simulink model "full_subtractor"  (R2021a)
settings: Solver=VariableStepAuto  StartTime=0.0  StopTime=10.0  RelTol=1e-3
settings Model: Creator=kbhar  LastModifiedBy=kbhar

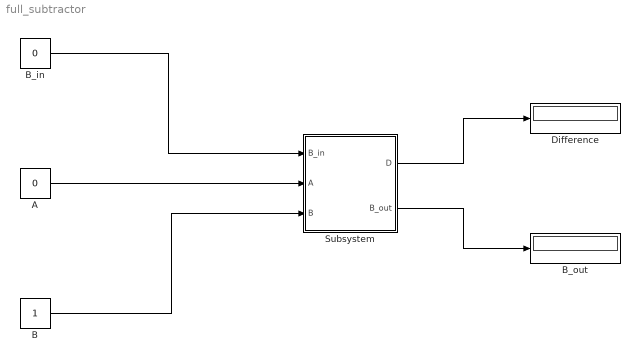
== system full_subtractor ==
  A : Constant  Value=0
  B : Constant
  B_in : Constant  Value=0
  B_out : Display
  Difference : Display
  Subsystem : Subsystem
  wires:
  B_in/1 -> Subsystem/1(B_in)
  A/1 -> Subsystem/2(A)
  B/1 -> Subsystem/3(B)
  Subsystem/1(D) -> Difference/1
  Subsystem/2(B_out) -> B_out/1

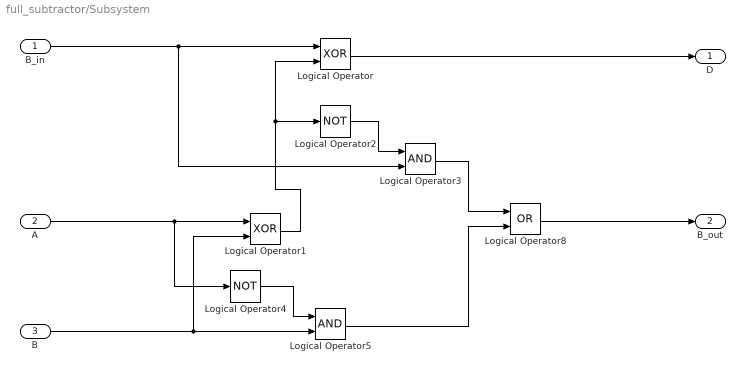
== system full_subtractor/Subsystem ==
  B_in : Inport
  A : Inport  Port=2
  B : Inport  Port=3
  Logical Operator : Logic  Operator=XOR  AllPortsSameDT=off  OutDataTypeStr=boolean
  Logical Operator1 : Logic  Operator=XOR  AllPortsSameDT=off  OutDataTypeStr=boolean
  Logical Operator2 : Logic  Operator=NOT  AllPortsSameDT=off  OutDataTypeStr=boolean
  Logical Operator3 : Logic  AllPortsSameDT=off  OutDataTypeStr=boolean
  Logical Operator4 : Logic  Operator=NOT  AllPortsSameDT=off  OutDataTypeStr=boolean
  Logical Operator5 : Logic  AllPortsSameDT=off  OutDataTypeStr=boolean
  Logical Operator8 : Logic  Operator=OR  AllPortsSameDT=off  OutDataTypeStr=boolean
  D : Outport
  B_out : Outport  Port=2
  wires:
  Logical Operator2/1 -> Logical Operator3/1
  B_in/1 -> Logical Operator/1, Logical Operator3/2
  B/1 -> Logical Operator1/2, Logical Operator5/2
  Logical Operator1/1 -> Logical Operator2/1, Logical Operator/2
  A/1 -> Logical Operator1/1, Logical Operator4/1
  Logical Operator3/1 -> Logical Operator8/1
  Logical Operator5/1 -> Logical Operator8/2
  Logical Operator4/1 -> Logical Operator5/1
  Logical Operator/1 -> D/1
  Logical Operator8/1 -> B_out/1
